simulink library "ACCA_lib"  (Simulink 7.5)
settings: Solver=ode45  StartTime=0.0  StopTime=10.0  RelTol=1e-3
values from neighbouring files (symbols this model uses):
  pACCA_bool_KickDwnSel_C = Simulink.Parameter    [ACCA_par.m]
  pACCA_kmph_AccPedVehSpdMax_C = Simulink.Parameter    [ACCA_par.m]
  pACCA_kmph_AccPedVehSpdMin_C = Simulink.Parameter    [ACCA_par.m]
  pACCA_Nm_AccPedDrvTrqMax_C = Simulink.Parameter    [ACCA_par.m]
  pACCA_Nm_AccPedDrvTrqMin_C = Simulink.Parameter    [ACCA_par.m]
  pACCA_Nm_DrvTrqZero_C = Simulink.Parameter    [ACCA_par.m]
  pACCA_pct_AccPedMax_C = Simulink.Parameter    [ACCA_par.m]
  pACCA_pct_AccPedMin_C = Simulink.Parameter    [ACCA_par.m]
  pACCA_pct_KickDwnLoAccPed_C = Simulink.Parameter    [ACCA_par.m]
  pACCA_pct_KickDwnUpAccPed_C = Simulink.Parameter    [ACCA_par.m]
  pACCA_pct_OverrideOutAccPed_C = Simulink.Parameter    [ACCA_par.m]
  pACCA_pct_VirAccPed_MAP = Simulink.Parameter    [ACCA_par.m]
  pACCA_s_ACCBtnErrIdfyTi_C = Simulink.Parameter    [ACCA_par.m]
undefined symbols (not defined in the file or in its folder): ACCBtnStTyp, ACCStTyp, DiscIntNeverNeededParam, p_bool_False_M
libraries: BaseOperationLib_Browser x43
settings Model: Creator=wuaibin  LastModifiedBy=wuaibin

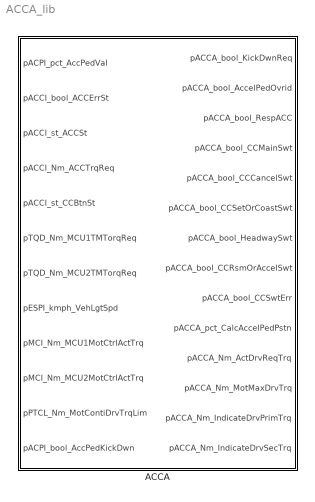
== system ACCA_lib ==
  ACCA : Subsystem

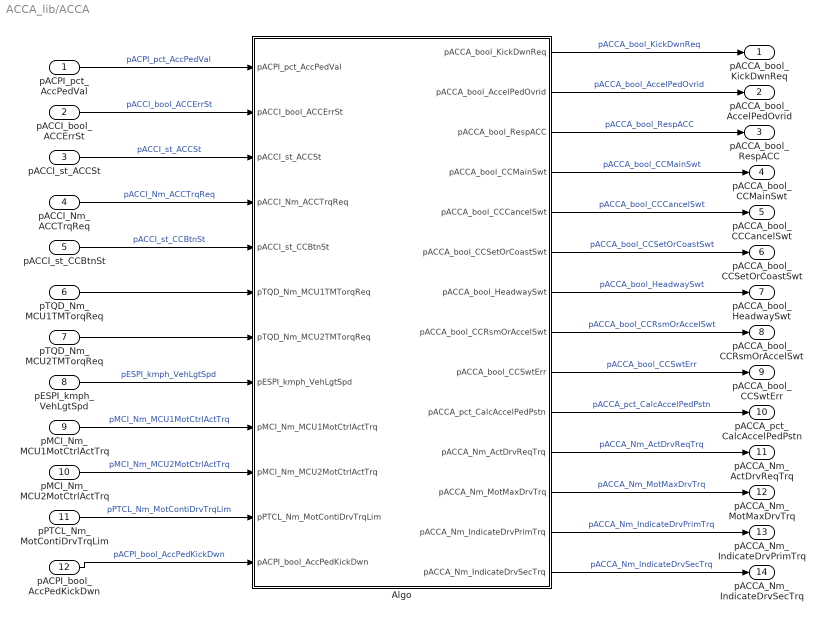
== system ACCA_lib/ACCA ==
  pACPI_pct_AccPedVal : Inport  OutDataType=fixdt(1, 16)  OutScaling=2^0
  pACCI_bool_ACCErrSt : Inport  Port=2  OutDataType=fixdt(1, 16)  OutScaling=2^0
  pACCI_st_ACCSt : Inport  Port=3  OutDataType=fixdt(1, 16)  OutScaling=2^0
  pACCI_Nm_ACCTrqReq : Inport  Port=4  OutDataType=fixdt(1, 16)  OutScaling=2^0
  pACCI_st_CCBtnSt : Inport  Port=5  OutDataType=fixdt(1, 16)  OutScaling=2^0
  pTQD_Nm_MCU1TMTorqReq : Inport  Port=6  OutDataType=fixdt(1, 16)  OutScaling=2^0
  pTQD_Nm_MCU2TMTorqReq : Inport  Port=7  OutDataType=fixdt(1, 16)  OutScaling=2^0
  pESPI_kmph_VehLgtSpd : Inport  Port=8  OutDataType=fixdt(1, 16)  OutScaling=2^0
  pMCI_Nm_MCU1MotCtrlActTrq : Inport  Port=9
  pMCI_Nm_MCU2MotCtrlActTrq : Inport  Port=10
  pPTCL_Nm_MotContiDrvTrqLim : Inport  Port=11
  pACPI_bool_AccPedKickDwn : Inport  Port=12
  Algo : Subsystem
  pACCA_bool_KickDwnReq : Outport  OutDataType=fixdt(1, 16)  OutScaling=2^0
  pACCA_bool_AccelPedOvrid : Outport  Port=2  OutDataType=fixdt(1, 16)  OutScaling=2^0
  pACCA_bool_RespACC : Outport  Port=3  OutDataType=fixdt(1, 16)  OutScaling=2^0
  pACCA_bool_CCMainSwt : Outport  Port=4
  pACCA_bool_CCCancelSwt : Outport  Port=5
  pACCA_bool_CCSetOrCoastSwt : Outport  Port=6
  pACCA_bool_HeadwaySwt : Outport  Port=7
  pACCA_bool_CCRsmOrAccelSwt : Outport  Port=8
  pACCA_bool_CCSwtErr : Outport  Port=9
  pACCA_pct_CalcAccelPedPstn : Outport  Port=10
  pACCA_Nm_ActDrvReqTrq : Outport  Port=11
  pACCA_Nm_MotMaxDrvTrq : Outport  Port=12
  pACCA_Nm_IndicateDrvPrimTrq : Outport  Port=13
  pACCA_Nm_IndicateDrvSecTrq : Outport  Port=14
  wires:
  Algo/13(pACCA_Nm_IndicateDrvPrimTrq) -> pACCA_Nm_IndicateDrvPrimTrq/1  "pACCA_Nm_IndicateDrvPrimTrq"
  Algo/12(pACCA_Nm_MotMaxDrvTrq) -> pACCA_Nm_MotMaxDrvTrq/1  "pACCA_Nm_MotMaxDrvTrq"
  Algo/11(pACCA_Nm_ActDrvReqTrq) -> pACCA_Nm_ActDrvReqTrq/1  "pACCA_Nm_ActDrvReqTrq"
  pPTCL_Nm_MotContiDrvTrqLim/1 -> Algo/11(pPTCL_Nm_MotContiDrvTrqLim)  "pPTCL_Nm_MotContiDrvTrqLim"
  pMCI_Nm_MCU2MotCtrlActTrq/1 -> Algo/10(pMCI_Nm_MCU2MotCtrlActTrq)  "pMCI_Nm_MCU2MotCtrlActTrq"
  pMCI_Nm_MCU1MotCtrlActTrq/1 -> Algo/9(pMCI_Nm_MCU1MotCtrlActTrq)  "pMCI_Nm_MCU1MotCtrlActTrq"
  Algo/10(pACCA_pct_CalcAccelPedPstn) -> pACCA_pct_CalcAccelPedPstn/1  "pACCA_pct_CalcAccelPedPstn"
  Algo/9(pACCA_bool_CCSwtErr) -> pACCA_bool_CCSwtErr/1  "pACCA_bool_CCSwtErr"
  Algo/8(pACCA_bool_CCRsmOrAccelSwt) -> pACCA_bool_CCRsmOrAccelSwt/1  "pACCA_bool_CCRsmOrAccelSwt"
  Algo/7(pACCA_bool_HeadwaySwt) -> pACCA_bool_HeadwaySwt/1  "pACCA_bool_HeadwaySwt"
  Algo/6(pACCA_bool_CCSetOrCoastSwt) -> pACCA_bool_CCSetOrCoastSwt/1  "pACCA_bool_CCSetOrCoastSwt"
  Algo/5(pACCA_bool_CCCancelSwt) -> pACCA_bool_CCCancelSwt/1  "pACCA_bool_CCCancelSwt"
  Algo/4(pACCA_bool_CCMainSwt) -> pACCA_bool_CCMainSwt/1  "pACCA_bool_CCMainSwt"
  Algo/3(pACCA_bool_RespACC) -> pACCA_bool_RespACC/1  "pACCA_bool_RespACC"
  Algo/2(pACCA_bool_AccelPedOvrid) -> pACCA_bool_AccelPedOvrid/1  "pACCA_bool_AccelPedOvrid"
  Algo/1(pACCA_bool_KickDwnReq) -> pACCA_bool_KickDwnReq/1  "pACCA_bool_KickDwnReq"
  pESPI_kmph_VehLgtSpd/1 -> Algo/8(pESPI_kmph_VehLgtSpd)  "pESPI_kmph_VehLgtSpd"
  pACCI_st_CCBtnSt/1 -> Algo/5(pACCI_st_CCBtnSt)  "pACCI_st_CCBtnSt"
  pACCI_Nm_ACCTrqReq/1 -> Algo/4(pACCI_Nm_ACCTrqReq)  "pACCI_Nm_ACCTrqReq"
  pACCI_st_ACCSt/1 -> Algo/3(pACCI_st_ACCSt)  "pACCI_st_ACCSt"
  pACCI_bool_ACCErrSt/1 -> Algo/2(pACCI_bool_ACCErrSt)  "pACCI_bool_ACCErrSt"
  pACPI_pct_AccPedVal/1 -> Algo/1(pACPI_pct_AccPedVal)  "pACPI_pct_AccPedVal"
  pACPI_bool_AccPedKickDwn/1 -> Algo/12(pACPI_bool_AccPedKickDwn)  "pACPI_bool_AccPedKickDwn"
  Algo/14(pACCA_Nm_IndicateDrvSecTrq) -> pACCA_Nm_IndicateDrvSecTrq/1  "pACCA_Nm_IndicateDrvSecTrq"
  pTQD_Nm_MCU1TMTorqReq/1 -> Algo/6(pTQD_Nm_MCU1TMTorqReq)
  pTQD_Nm_MCU2TMTorqReq/1 -> Algo/7(pTQD_Nm_MCU2TMTorqReq)

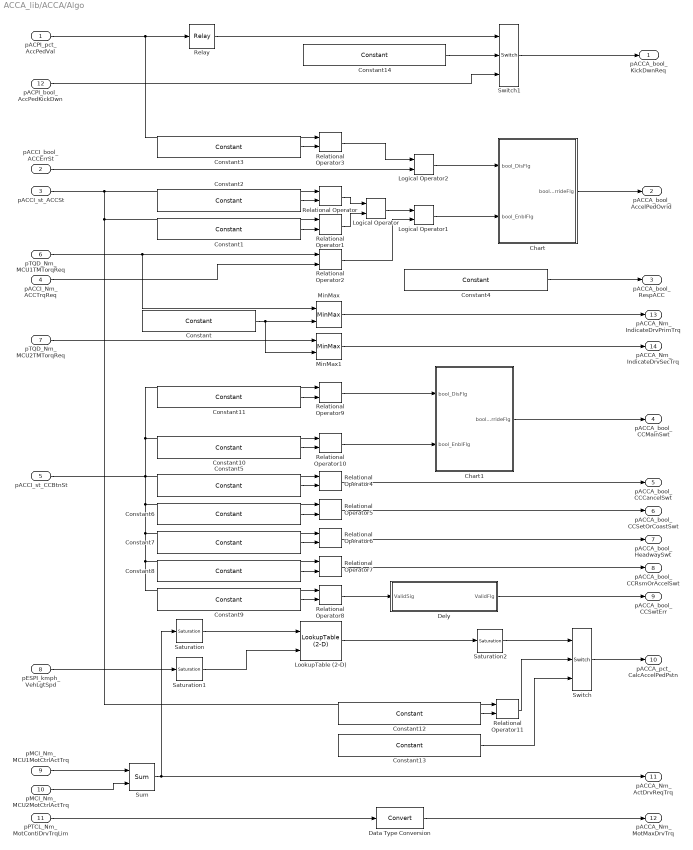
== system ACCA_lib/ACCA/Algo ==
  pACPI_pct_AccPedVal : Inport  OutDataType=fixdt(1, 16)  OutScaling=2^0
  pACCI_bool_ACCErrSt : Inport  Port=2  OutDataType=fixdt(1, 16)  OutScaling=2^0
  pACCI_st_ACCSt : Inport  Port=3  OutDataType=fixdt(1, 16)  OutScaling=2^0
  pACCI_Nm_ACCTrqReq : Inport  Port=4  OutDataType=fixdt(1, 16)  OutScaling=2^0
  pACCI_st_CCBtnSt : Inport  Port=5  OutDataType=fixdt(1, 16)  OutScaling=2^0
  pTQD_Nm_MCU1TMTorqReq : Inport  Port=6  OutDataType=fixdt(1, 16)  OutScaling=2^0
  pTQD_Nm_MCU2TMTorqReq : Inport  Port=7  OutDataType=fixdt(1, 16)  OutScaling=2^0
  pESPI_kmph_VehLgtSpd : Inport  Port=8  OutDataType=fixdt(1, 16)  OutScaling=2^0
  pMCI_Nm_MCU1MotCtrlActTrq : Inport  Port=9  OutDataType=fixdt(1, 16)  OutScaling=2^0
  pMCI_Nm_MCU2MotCtrlActTrq : Inport  Port=10  OutDataType=fixdt(1, 16)  OutScaling=2^0
  pPTCL_Nm_MotContiDrvTrqLim : Inport  Port=11  OutDataType=fixdt(1, 16)  OutScaling=2^0
  pACPI_bool_AccPedKickDwn : Inport  Port=12  OutDataType=fixdt(1, 16)  OutScaling=2^0
  Chart : Stateflow chart  TreatAsAtomicUnit=on
  Chart1 : Stateflow chart  TreatAsAtomicUnit=on
  Constant : BaseOperationLib_Browser/Sources&Sinks/Constant  Value=pACCA_Nm_DrvTrqZero_C  OutMin=[]  OutMax=[]  OutDataType=fixdt(1, 16)  ConRadixGroup=Use specified scaling  OutScaling=2^0  OutDataTypeStr=Inherit: Inherit from 'Constant value'
  Constant1 : BaseOperationLib_Browser/Sources&Sinks/Constant  Value=uint8(ACCStTyp.ACCST_Override)  OutMin=[]  OutMax=[]  OutDataType=Enum: ACCStTyp  ConRadixGroup=Best Precision: Vector-wise  OutScaling=[]  OutDataTypeStr=Inherit: Inherit from 'Constant value'
  Constant10 : BaseOperationLib_Browser/Sources&Sinks/Constant  Value=uint8(ACCBtnStTyp.ACCBST_MainOn)  OutMin=[]  OutMax=[]  OutDataType=Enum: ACCStTyp  ConRadixGroup=Best Precision: Vector-wise  OutScaling=[]  OutDataTypeStr=Inherit: Inherit from 'Constant value'
  Constant11 : BaseOperationLib_Browser/Sources&Sinks/Constant  Value=uint8(ACCBtnStTyp.ACCBST_MainOff)  OutMin=[]  OutMax=[]  OutDataType=Enum: ACCStTyp  ConRadixGroup=Best Precision: Vector-wise  OutScaling=[]  OutDataTypeStr=Inherit: Inherit from 'Constant value'
  Constant12 : BaseOperationLib_Browser/Sources&Sinks/Constant  Value=uint8(ACCStTyp.ACCST_Active)  OutMin=[]  OutMax=[]  OutDataType=Enum: ACCStTyp  ConRadixGroup=Best Precision: Vector-wise  OutScaling=[]  OutDataTypeStr=Inherit: Inherit from 'Constant value'
  Constant13 : BaseOperationLib_Browser/Sources&Sinks/Constant  Value=pACCA_pct_AccPedMin_C  OutMin=[]  OutMax=[]  OutDataType=Enum: ACCStTyp  ConRadixGroup=Best Precision: Vector-wise  OutScaling=[]  OutDataTypeStr=Inherit: Inherit from 'Constant value'
  Constant14 : BaseOperationLib_Browser/Sources&Sinks/Constant  Value=pACCA_bool_KickDwnSel_C  OutMin=[]  OutMax=[]  OutDataType=Enum: ACCStTyp  ConRadixGroup=Best Precision: Vector-wise  OutScaling=[]  OutDataTypeStr=Inherit: Inherit from 'Constant value'
  Constant2 : BaseOperationLib_Browser/Sources&Sinks/Constant  Value=uint8(ACCStTyp.ACCST_Active)  OutMin=[]  OutMax=[]  OutDataType=Enum: ACCStTyp  ConRadixGroup=Best Precision: Vector-wise  OutScaling=[]  OutDataTypeStr=Inherit: Inherit from 'Constant value'
  Constant3 : BaseOperationLib_Browser/Sources&Sinks/Constant  Value=pACCA_pct_OverrideOutAccPed_C  OutMin=[]  OutMax=[]  OutDataType=Enum: ACCStTyp  ConRadixGroup=Best Precision: Vector-wise  OutScaling=[]  OutDataTypeStr=Inherit: Inherit from 'Constant value'
  Constant4 : BaseOperationLib_Browser/Sources&Sinks/Constant  Value=p_bool_False_M  OutMin=[]  OutMax=[]  OutDataType=Enum: ACCStTyp  ConRadixGroup=Best Precision: Vector-wise  OutScaling=[]  OutDataTypeStr=Inherit: Inherit from 'Constant value'
  Constant5 : BaseOperationLib_Browser/Sources&Sinks/Constant  Value=uint8(ACCBtnStTyp.ACCBST_Cancel)  OutMin=[]  OutMax=[]  OutDataType=Enum: ACCStTyp  ConRadixGroup=Best Precision: Vector-wise  OutScaling=[]  OutDataTypeStr=Inherit: Inherit from 'Constant value'
  Constant6 : BaseOperationLib_Browser/Sources&Sinks/Constant  Value=uint8(ACCBtnStTyp.ACCBST_Set)  OutMin=[]  OutMax=[]  OutDataType=Enum: ACCStTyp  ConRadixGroup=Best Precision: Vector-wise  OutScaling=[]  OutDataTypeStr=Inherit: Inherit from 'Constant value'
  Constant7 : BaseOperationLib_Browser/Sources&Sinks/Constant  Value=uint8(ACCBtnStTyp.ACCBST_Headway)  OutMin=[]  OutMax=[]  OutDataType=Enum: ACCStTyp  ConRadixGroup=Best Precision: Vector-wise  OutScaling=[]  OutDataTypeStr=Inherit: Inherit from 'Constant value'
  Constant8 : BaseOperationLib_Browser/Sources&Sinks/Constant  Value=uint8(ACCBtnStTyp.ACCBST_Resume)  OutMin=[]  OutMax=[]  OutDataType=Enum: ACCStTyp  ConRadixGroup=Best Precision: Vector-wise  OutScaling=[]  OutDataTypeStr=Inherit: Inherit from 'Constant value'
  Constant9 : BaseOperationLib_Browser/Sources&Sinks/Constant  Value=uint8(ACCBtnStTyp.ACCBST_Fault)  OutMin=[]  OutMax=[]  OutDataType=Enum: ACCStTyp  ConRadixGroup=Best Precision: Vector-wise  OutScaling=[]  OutDataTypeStr=Inherit: Inherit from 'Constant value'
  Data Type Conversion : DataTypeConversion  OutDataType=fixdt(1, 16)  OutScaling=2^0
  Dely : Subsystem  mask{timeoutthres=pACCA_s_ACCBtnErrIdfyTi_C}
      mask prompts: timeoutthres "Timeout counter Treshold"
      mask help:
      | WatchDog block
      |
      | If input bool signal is false for the number of step bigger than "Timeout counter Threshold" the output WatchDog signal is set to True.
      |
      | Tip. Set the thresshold to the required time in seconds devided by algorithm sampling time.
      mask Help:
      | WatchDog block
      | 
      | If input bool signal is false for the number of step bigger than "Timeout counter Threshold" the output WatchDog signal is set to True.
      | 
      | Tip. Set the thresshold to required time in second devided by sampling time.
  Logical Operator : BaseOperationLib_Browser/Logic Operations Changed/Logical Operator  Operator=OR  Inputs=2  AllPortsSameDT=on  OutDataTypeMode=Specify via dialog  LogicDataType=PDT_Bool  OutDataTypeStr=PDT_Bool
  Logical Operator1 : BaseOperationLib_Browser/Logic Operations Changed/Logical Operator  Operator=AND  Inputs=2  AllPortsSameDT=on  OutDataTypeMode=Specify via dialog  LogicDataType=PDT_Bool  OutDataTypeStr=PDT_Bool
  Logical Operator2 : BaseOperationLib_Browser/Logic Operations Changed/Logical Operator  Operator=OR  Inputs=2  AllPortsSameDT=on  OutDataTypeMode=Specify via dialog  LogicDataType=PDT_Bool  OutDataTypeStr=PDT_Bool
  LookupTable (2-D) : BaseOperationLib_Browser/Lookup Tables Changed/LookupTable (2-D)  RowIndex=pACCA_Nm_AccPedDrvTrq_TABX  ColumnIndex=pACCA_kmph_AccPedVehSpd_TABY  Table=pACCA_pct_VirAccPed_MAP  LookUpMeth=Interpolation-Use End Values  OutMin=[]  OutMax=[]  OutDataType=fixdt(1, 16)  OutScaling=2^0  OutDataTypeStr=Inherit: Inherit via back propagation  SaturateOnIntegerOverflow=on
      settings: AttributesFormatString=X:%<RowIndex>\nY:%<ColumnIndex>\nTAB:%<Table>
  MinMax : BaseOperationLib_Browser/Math Operations Changed/MinMax  Function=max  Inputs=2  InputSameDT=on  OutMin=[]  OutMax=[]  OutDataType=fixdt(1, 16)  OutScaling=2^0  SaturateOnIntegerOverflow=on
  MinMax1 : BaseOperationLib_Browser/Math Operations Changed/MinMax  Function=max  Inputs=2  InputSameDT=on  OutMin=[]  OutMax=[]  OutDataType=fixdt(1, 16)  OutScaling=2^0  SaturateOnIntegerOverflow=on
  Relational Operator{,1,4..11} (10 alike) : BaseOperationLib_Browser/Logic Operations Changed/Relational Operator  Operator===  InputSameDT=on  LogicOutDataTypeMode=Specify via dialog  LogicDataType=PDT_Bool  OutDataTypeStr=PDT_Bool
  Relational Operator2 : BaseOperationLib_Browser/Logic Operations Changed/Relational Operator  Operator=>  InputSameDT=on  LogicOutDataTypeMode=Specify via dialog  LogicDataType=PDT_Bool  OutDataTypeStr=PDT_Bool
  Relational Operator3 : BaseOperationLib_Browser/Logic Operations Changed/Relational Operator  Operator=<=  InputSameDT=on  LogicOutDataTypeMode=Specify via dialog  LogicDataType=PDT_Bool  OutDataTypeStr=PDT_Bool
  Relay : BaseOperationLib_Browser/Discontinuities Changed/Relay  OnSwitchValue=pACCA_pct_KickDwnUpAccPed_C  OffSwitchValue=pACCA_pct_KickDwnLoAccPed_C  OnOutputValue=p_bool_True_M  OffOutputValue=p_bool_False_M  OutMin=[]  OutMax=[]  OutDataType=fixdt(1, 16)  ConRadixGroup=Use specified scaling  OutScaling=2^0  OutDataTypeStr=Inherit: Inherit via back propagation
      settings: AttributesFormatString=%<OnSwitchValue> OnOut %<OnOutputValue>\n%<OffSwitchValue> OffOut %<OffOutputValue>
  Saturation : BaseOperationLib_Browser/Discontinuities Unchanged/Saturation  UpperLimit=pACCA_Nm_AccPedDrvTrqMax_C  LowerLimit=pACCA_Nm_AccPedDrvTrqMin_C  OutMin=[]  OutMax=[]  OutDataType=fixdt(1, 16)  OutScaling=2^0
      settings: AttributesFormatString=ULim:%<UpperLimit>\nLLim:%<LowerLimit>
  Saturation1 : BaseOperationLib_Browser/Discontinuities Unchanged/Saturation  UpperLimit=pACCA_kmph_AccPedVehSpdMax_C  LowerLimit=pACCA_kmph_AccPedVehSpdMin_C  OutMin=[]  OutMax=[]  OutDataType=fixdt(1, 16)  OutScaling=2^0
      settings: AttributesFormatString=ULim:%<UpperLimit>\nLLim:%<LowerLimit>
  Saturation2 : BaseOperationLib_Browser/Discontinuities Unchanged/Saturation  UpperLimit=pACCA_pct_AccPedMax_C  LowerLimit=pACCA_pct_AccPedMin_C  OutMin=[]  OutMax=[]  OutDataType=fixdt(1, 16)  OutScaling=2^0
      settings: AttributesFormatString=ULim:%<UpperLimit>\nLLim:%<LowerLimit>
  Sum : BaseOperationLib_Browser/Math Operations Changed/Sum  Inputs=++  InputSameDT=on  OutMin=[]  OutMax=[]  OutDataType=fixdt(1, 16)  OutScaling=2^0  SaturateOnIntegerOverflow=on
  Switch : BaseOperationLib_Browser/Signal Routing Changed/Switch  Criteria=u2 ~= 0  Threshold=1  InputSameDT=on  OutMin=[]  OutMax=[]  OutDataType=fixdt(1,16,0)  OutScaling=[]  SaturateOnIntegerOverflow=on
  Switch1 : BaseOperationLib_Browser/Signal Routing Changed/Switch  Criteria=u2 ~= 0  Threshold=1  InputSameDT=on  OutMin=[]  OutMax=[]  OutDataType=fixdt(1,16,0)  OutScaling=[]  SaturateOnIntegerOverflow=on
  pACCA_bool_KickDwnReq : Outport  OutDataType=fixdt(1, 16)  OutScaling=2^0
  pACCA_bool_AccelPedOvrid : Outport  Port=2  OutDataType=fixdt(1, 16)  OutScaling=2^0
  pACCA_bool_RespACC : Outport  Port=3  OutDataType=fixdt(1, 16)  OutScaling=2^0
  pACCA_bool_CCMainSwt : Outport  Port=4
  pACCA_bool_CCCancelSwt : Outport  Port=5
  pACCA_bool_CCSetOrCoastSwt : Outport  Port=6
  pACCA_bool_HeadwaySwt : Outport  Port=7
  pACCA_bool_CCRsmOrAccelSwt : Outport  Port=8
  pACCA_bool_CCSwtErr : Outport  Port=9
  pACCA_pct_CalcAccelPedPstn : Outport  Port=10
  pACCA_Nm_ActDrvReqTrq : Outport  Port=11
  pACCA_Nm_MotMaxDrvTrq : Outport  Port=12
  pACCA_Nm_IndicateDrvPrimTrq : Outport  Port=13
  pACCA_Nm_IndicateDrvSecTrq : Outport  Port=14
  wires:
  Constant13/1 -> Switch/3
  Constant12/1 -> Relational Operator11/2
  Relational Operator11/1 -> Switch/2
  Switch/1 -> pACCA_pct_CalcAccelPedPstn/1
  Saturation2/1 -> Switch/1
  Data Type Conversion/1 -> pACCA_Nm_MotMaxDrvTrq/1
  MinMax/1 -> pACCA_Nm_IndicateDrvPrimTrq/1
  Constant/1 -> MinMax/2, MinMax1/2
  pPTCL_Nm_MotContiDrvTrqLim/1 -> Data Type Conversion/1
  Sum/1 -> Saturation/1, pACCA_Nm_ActDrvReqTrq/1
  pMCI_Nm_MCU2MotCtrlActTrq/1 -> Sum/2
  pMCI_Nm_MCU1MotCtrlActTrq/1 -> Sum/1
  pTQD_Nm_MCU1TMTorqReq/1 -> MinMax/1, Relational Operator2/1
  LookupTable (2-D)/1 -> Saturation2/1
  Saturation1/1 -> LookupTable (2-D)/2
  pESPI_kmph_VehLgtSpd/1 -> Saturation1/1
  Saturation/1 -> LookupTable (2-D)/1
  Constant11/1 -> Relational Operator9/2
  Constant10/1 -> Relational Operator10/2
  Chart1/1(bool_OverrideFlg) -> pACCA_bool_CCMainSwt/1
  Relational Operator10/1 -> Chart1/2(bool_EnblFlg)
  Relational Operator9/1 -> Chart1/1(bool_DisFlg)
  Dely/1(ValidFlg) -> pACCA_bool_CCSwtErr/1
  Relational Operator8/1 -> Dely/1(ValidSig)
  Relational Operator7/1 -> pACCA_bool_CCRsmOrAccelSwt/1
  Relational Operator6/1 -> pACCA_bool_HeadwaySwt/1
  Relational Operator5/1 -> pACCA_bool_CCSetOrCoastSwt/1
  Relational Operator4/1 -> pACCA_bool_CCCancelSwt/1
  Constant9/1 -> Relational Operator8/2
  Constant8/1 -> Relational Operator7/2
  Constant7/1 -> Relational Operator6/2
  Constant6/1 -> Relational Operator5/2
  Constant5/1 -> Relational Operator4/2
  pACCI_st_CCBtnSt/1 -> Relational Operator10/1, Relational Operator9/1, Relational Operator8/1, Relational Operator7/1, Relational Operator6/1, Relational Operator5/1, Relational Operator4/1
  Constant4/1 -> pACCA_bool_RespACC/1
  Logical Operator2/1 -> Chart/1(bool_DisFlg)
  Relational Operator3/1 -> Logical Operator2/1
  Constant3/1 -> Relational Operator3/2
  Chart/1(bool_OverrideFlg) -> pACCA_bool_AccelPedOvrid/1
  pACCI_bool_ACCErrSt/1 -> Logical Operator2/2
  Logical Operator1/1 -> Chart/2(bool_EnblFlg)
  Relational Operator2/1 -> Logical Operator1/2
  pACCI_Nm_ACCTrqReq/1 -> Relational Operator2/2
  Logical Operator/1 -> Logical Operator1/1
  Relational Operator1/1 -> Logical Operator/2
  Relational Operator/1 -> Logical Operator/1
  Constant1/1 -> Relational Operator1/2
  Constant2/1 -> Relational Operator/2
  pACCI_st_ACCSt/1 -> Relational Operator11/1, Relational Operator1/1, Relational Operator/1
  pACPI_pct_AccPedVal/1 -> Relational Operator3/1, Relay/1
  Switch1/1 -> pACCA_bool_KickDwnReq/1
  Relay/1 -> Switch1/1
  pACPI_bool_AccPedKickDwn/1 -> Switch1/3
  Constant14/1 -> Switch1/2
  MinMax1/1 -> pACCA_Nm_IndicateDrvSecTrq/1
  pTQD_Nm_MCU2TMTorqReq/1 -> MinMax1/1

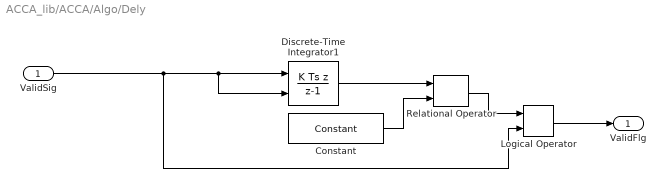
== system ACCA_lib/ACCA/Algo/Dely ==
  ValidSig : Inport  OutDataType=fixdt(1, 16)  OutScaling=2^0
  Constant : BaseOperationLib_Browser/Sources&Sinks/Constant  Value=timeoutthres  OutMin=[]  OutMax=[]  OutDataType=fixdt(1, 16)  ConRadixGroup=Use specified scaling  OutScaling=2^0  OutDataTypeStr=Inherit: Inherit from 'Constant value'
  Discrete-Time Integrator1 : DiscreteIntegrator  IntegratorMethod=Integration: Backward Euler  ExternalReset=rising  SampleTime=-1  OutDataType=PDT_s  OutDataTypeStr=Inherit: Inherit via back propagation  UpperSaturationLimit=100  LowerSaturationLimit=0  ICPrevOutput=DiscIntNeverNeededParam  ICPrevScaledInput=DiscIntNeverNeededParam
  Logical Operator : BaseOperationLib_Browser/Logic Operations Changed/Logical Operator  Operator=AND  Inputs=2  AllPortsSameDT=on  OutDataTypeMode=Specify via dialog  LogicDataType=PDT_Bool  OutDataTypeStr=PDT_Bool
  Relational Operator : BaseOperationLib_Browser/Logic Operations Changed/Relational Operator  Operator=>=  InputSameDT=on  LogicOutDataTypeMode=Specify via dialog  LogicDataType=PDT_Bool  OutDataTypeStr=PDT_Bool
  ValidFlg : Outport  OutDataType=fixdt(1, 16)  OutScaling=2^0
  wires:
  Discrete-Time Integrator1/1 -> Relational Operator/1
  Constant/1 -> Relational Operator/2
  Logical Operator/1 -> ValidFlg/1
  Relational Operator/1 -> Logical Operator/1
  ValidSig/1 -> Logical Operator/2, Discrete-Time Integrator1/2, Discrete-Time Integrator1/1

== stateflow chart ACCA/Algo/Chart ==
  state Normal
    en:
    bool_OverrideFlg=false;
  state Override
    en:
    bool_OverrideFlg=true;
  (default) -> Normal
  Normal -> Override : [bool_EnblFlg==true]
  Override -> Normal : [bool_DisFlg==true]
  data: bool_DisFlg input double; bool_EnblFlg input double; bool_OverrideFlg output boolean

== stateflow chart ACCA/Algo/Chart1 ==
  state Normal
    en:
    bool_OverrideFlg=false;
  state Override
    en:
    bool_OverrideFlg=true;
  (default) -> Normal
  Normal -> Override : [bool_EnblFlg==true]
  Override -> Normal : [bool_DisFlg==true]
  data: bool_DisFlg input double; bool_EnblFlg input double; bool_OverrideFlg output boolean
